simulink model "test_buck_pid"  (R2019a)
settings: Solver=ode8  StartTime=0.0  StopTime=2  RelTol=1e-3  EnableMultiTasking=on
values from neighbouring files (symbols this model uses):
  a00c = sys(1).Ac(1,1)    [controller_comparison.m]
  a00o = -rL/L    (= -196.226415094)    [controller_comparison.m]
  a01c = sys(1).Ac(1,2)    [controller_comparison.m]
  a01o = sys(1).Ac(1,2)    [controller_comparison.m]
  a10c = sys(1).Ac(2,1)    [controller_comparison.m]
  a10o = sys(1).Ac(2,1)    [controller_comparison.m]
  a11c = sys(1).Ac(2,2)    [controller_comparison.m]
  a11o = sys(1).Ac(2,2)    [controller_comparison.m]
  b0c = sys(1).Bc(1)    [controller_comparison.m]
  b0o = sys(1).Bo(1)    [controller_comparison.m]
  b1c = sys(1).Bc(2)    [controller_comparison.m]
  b1o = sys(1).Bo(2)    [controller_comparison.m]
  i0 = 0    [controller_comparison.m]
  T_sw = 1/10000    (= 0.0001)    [controller_comparison.m]
  v0 = 0    [controller_comparison.m]
  Vref = 10    [controller_comparison.m]
libraries: simulink x2
settings Model: Creator=Omar  LastModifiedBy=omar
settings DataIOCC: LimitDataPoints=on  SaveFormat=Array  SignalLoggingSaveFormat=ModelDataLogs  ReturnWorkspaceOutputs=off
settings OptimizationCC: ExpressionDepthLimit=2147483647  LifeSpan=inf
settings DebuggingCC: UnderspecifiedInitializationDetection=Classic  MergeDetectMultiDrivingBlocksExec=none  MaxConsecutiveZCsMsg=none  SolverPrmCheckMsg=warning  MultiTaskDSMMsg=warning  MultiTaskCondExecSysMsg=none  StateNameClashWarn=warning  SFUnexpectedBacktrackingDiag=warning  SFNoUnconditionalDefaultTransitionDiag=warning  SFExecutionAtInitializationDiag=none  ArithmeticOperatorsInVariantConditions=warning
settings HardwareCC: ProdBitPerPointer=32  ProdBitPerSizeT=32  ProdBitPerPtrDiffT=32  ProdLargestAtomicFloat=None  ProdIntDivRoundTo=Undefined  ProdEndianess=Unspecified  ProdWordSize=32  ProdHWDeviceType=32-bit Generic
settings ModelReferenceCC: PropagateSignalLabelsOutOfModel=off
settings SFSimCC: SimUseLocalCustomCode=off
settings RTWCC: RTWUseLocalCustomCode=off
settings CodeAppCC: StateflowObjectComments=on
settings GRTTargetCC: TargetLangStandard=C89/C90 (ANSI)  GeneratePreprocessorConditionals=Disable all
settings ConfigComp: CovMetricSettings=dw  CovHtmlReporting=on  CovSaveCumulativeToWorkspaceVar=on  CovSaveSingleToWorkspaceVar=on  CovExternalEMLEnable=off

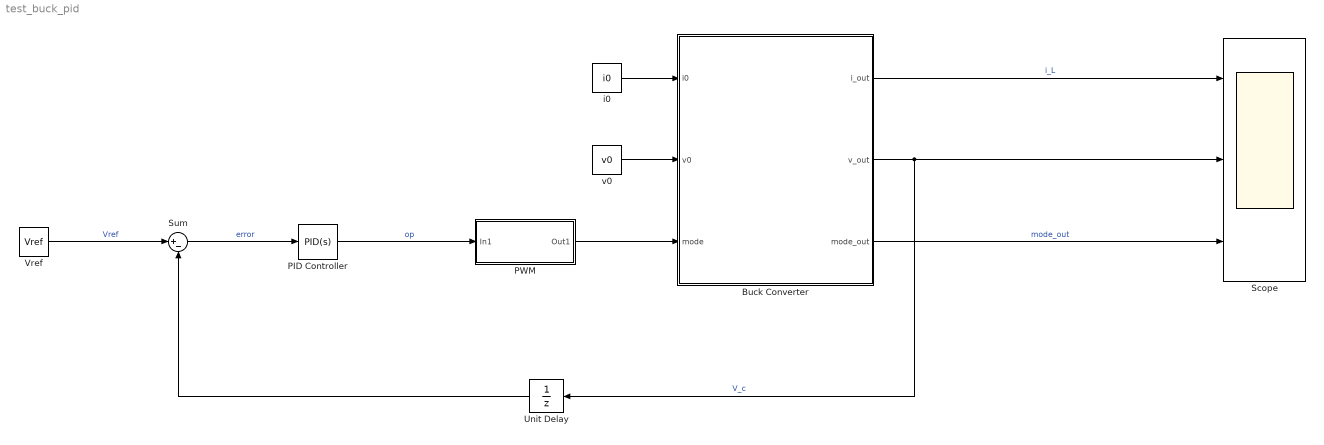
== system test_buck_pid ==
  Buck Converter : Stateflow chart  TreatAsAtomicUnit=on
  PID Controller : simulink/Continuous/PID Controller  Controller=PID  Form=Ideal  TimeDomain=Continuous-time  SampleTime=-1  IntegratorMethod=Forward Euler  FilterMethod=Forward Euler  ControllerParametersSource=internal  P=1.2  I=0.6  D=0.03  UseFilter=on  N=600  TunerSelectOption=Transfer Function Based (PID Tuner App)  InitialConditionSource=internal  InitialConditionForIntegrator=0  InitialConditionForFilter=0  DifferentiatorICPrevScaledInput=0  ExternalReset=none  TrackingMode=off  Kt=1  LimitOutput=off  UpperSaturationLimit=inf  LowerSaturationLimit=-inf  LinearizeAsGain=on  AntiWindupMode=none  Kb=1  POutMin=[]  POutMax=[]  IOutMin=[]  IOutMax=[]  DOutMin=[]  DOutMax=[]  NOutMin=[]  NOutMax=[]  SumOutMin=[]  SumOutMax=[]  SaturationOutMin=[]  SaturationOutMax=[]  PParamMin=[]  PParamMax=[]  IParamMin=[]  IParamMax=[]  DParamMin=[]  DParamMax=[]  NParamMin=[]  NParamMax=[]  KbParamMin=[]  KbParamMax=[]  KtParamMin=[]  KtParamMax=[]  KbOutMin=[]  KbOutMax=[]  KtOutMin=[]  KtOutMax=[]  IntegratorOutMin=[]  IntegratorOutMax=[]  FilterOutMin=[]  FilterOutMax=[]  SumI1OutMin=[]  SumI1OutMax=[]  SumI2OutMin=[]  SumI2OutMax=[]  SumI3OutMin=[]  SumI3OutMax=[]  SumI4OutMin=[]  SumI4OutMax=[]  SumDOutMin=[]  SumDOutMax=[]  DifferentiatorOutMin=[]  DifferentiatorOutMax=[]  FilterDiffOutCoefMin=[]  FilterDiffOutCoefMax=[]  ReciprocalOutMin=[]  ReciprocalOutMax=[]  SumDenOutMin=[]  SumDenOutMax=[]  SumNumOutMin=[]  SumNumOutMax=[]  DivideOutMin=[]  DivideOutMax=[]  IntegratorContinuousStateAttributes=''  IntegratorStateMustResolveToSignalObject=off  IntegratorRTWStateStorageClass=Auto  FilterContinuousStateAttributes=''  FilterStateMustResolveToSignalObject=off  FilterRTWStateStorageClass=Auto  ParallelPVariant=Passthrough  IdealPVariant=InternalParameters  IVariant=InternalParameters  DVariant=InternalParameters  IntegratorVariant=Continuous  SatVariant=Disabled  AWVariant=Passthrough  PCopyVariant=Disabled  TRVariant=Disabled  FdbkBlocksVariant=Forward  IdealPFdbkVariant=Disabled  SatFdbkVariant=Disabled  DerivativeFilterVariant=ContFilter  NVariant=InternalParameters  NCopyVariant=Disabled  FilterICVariant=InternalICsFilter  IntegratorICVariant=InternalICs  ExternalResetVariant=Disabled  TRSumVariant=Passthrough  SumFdbkVariant=Disabled  SumVariant=Sum_PID
  PWM : Subsystem
  Scope : Scope  NumInputPorts=3
  Sum : Sum  Inputs=|+-
  Unit Delay : UnitDelay  SampleTime=-1  HasFrameUpgradeWarning=on
  Vref : Constant  Value=Vref
  i0 : Constant  Value=i0
  v0 : Constant  Value=v0
  wires:
  Buck Converter/2(v_out) -> Unit Delay/1, Scope/2  "V_c"
  i0/1 -> Buck Converter/1(i0)
  v0/1 -> Buck Converter/2(v0)
  Buck Converter/3(mode_out) -> Scope/3  "mode_out"
  PWM/1(Out1) -> Buck Converter/3(mode)
  Unit Delay/1 -> Sum/2
  PID Controller/1 -> PWM/1(In1)  "op"
  Sum/1 -> PID Controller/1  "error"
  Vref/1 -> Sum/1  "Vref"
  Buck Converter/1(i_out) -> Scope/1  "i_L"

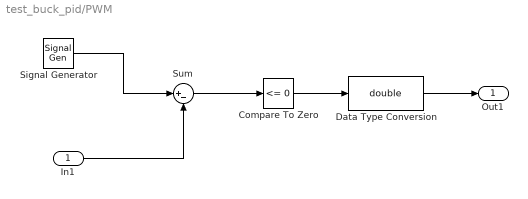
== system test_buck_pid/PWM ==
  In1 : Inport
  Compare To Zero : simulink/Logic and Bit Operations/Compare To Zero  relop=<=  OutDataTypeStr=boolean
  Data Type Conversion : DataTypeConversion  OutDataTypeStr=double
  Signal Generator : SignalGenerator  WaveForm=sawtooth  Frequency=1/T_sw
  Sum : Sum  Inputs=|+-
  Out1 : Outport
  wires:
  In1/1 -> Sum/2
  Signal Generator/1 -> Sum/1
  Sum/1 -> Compare To Zero/1
  Data Type Conversion/1 -> Out1/1
  Compare To Zero/1 -> Data Type Conversion/1

== stateflow chart test_buck_pid/Buck Converter ==
  settings: updateMethod=CONTINUOUS
  state Discontinuous
    du:
    i_dot = 0;
    v_dot = a11o*v+b1o;
    t_dot = 1;
    i_out = i;
    v_out = v;
    mode_out=3;
  state Charging
    du:
    i_dot = a00c*i+a01c*v+b0c;
    v_dot = a10c*i+a11c*v+b1c;
    t_dot = 1;
    i_out = i;
    v_out = v;
    mode_out=2;
  state Discharging
    du:
    i_dot = a00o*i+a01o*v+b0o;
    v_dot = a10o*i+a11o*v+b1o;
    t_dot = 1;
    i_out = i;
    v_out = v;
    mode_out=1;
  Discharging -> Discontinuous [order 2] : [i < 0]
  Discontinuous -> Charging : [mode >= 1]
      | {t = 0;}
  Charging -> Discharging : [mode < 1]
  Discharging -> Charging [order 1] : [mode >= 1]
      | {t = 0;}
  (default) -> Charging : {i = i0;
      | v = v0;}
  data: t local double; i_out output double; v_out output double; i local double; a00o local double =a00o; a01o local double =a01o; a10o local double =a10o; a11o local double =a11o; a00c local double =a00c; a01c local double =a01c; a10c local double =a10c; a11c local double =a11c; b0o local double =b0o; b1o local double =b1o; b0c local double =b0c; b1c local double =b1c; v local double; i0 input double; v0 input double; mode input double =120; mode_out output double
  data t settings: updateMethod=SF_CONTINUOUS_TIME_DATA
  data i settings: updateMethod=SF_CONTINUOUS_TIME_DATA
  data v settings: updateMethod=SF_CONTINUOUS_TIME_DATA
